simulink subsystem "Day2_Scenario_1"  (R2024a)
settings: Solver=VariableStepAuto  StartTime=0.0  StopTime=10.0  RelTol=1e-3
libraries: CarMaker4SL x2
settings Model: Creator=junhyung.cha  LastModifiedBy=User

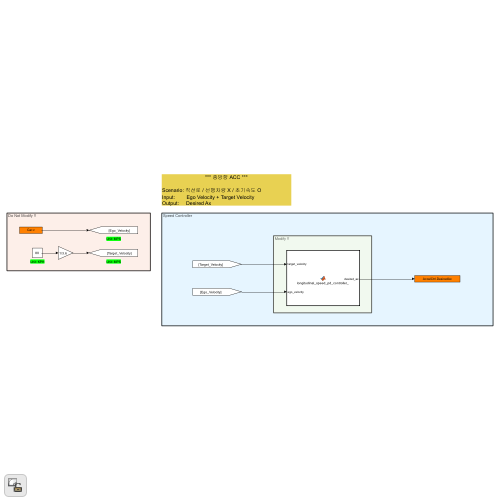
[thumbnail: Simulink's stored preview of the top-level diagram]
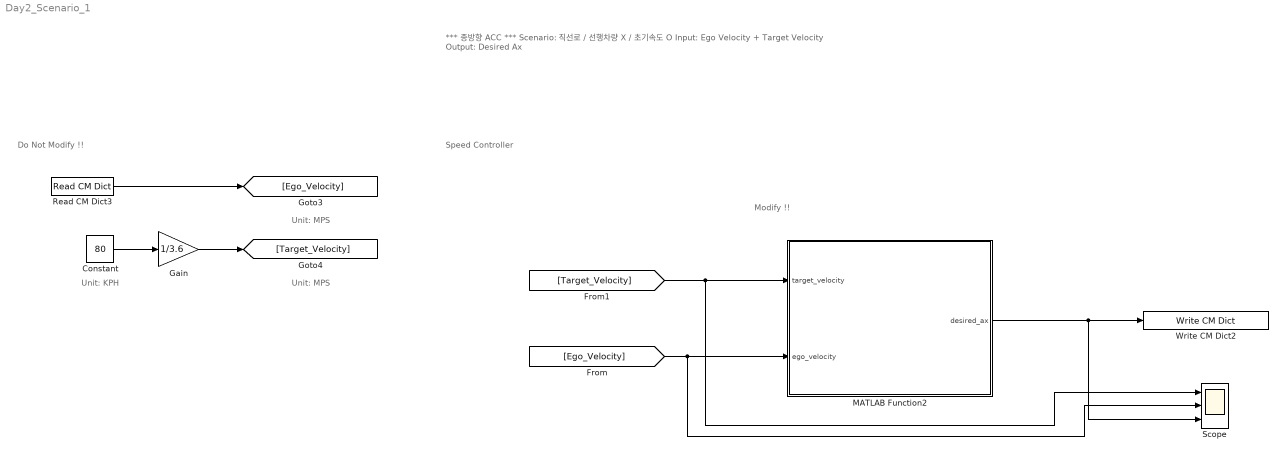
== system Day2_Scenario_1 ==
  note: Unit: KPH
  note: *** 종방향 ACC ***
      |
      | Scenario: 직선로 / 선행차량 X / 초기속도 O
      | Input: Ego Velocity + Target Velocity
      | Output: Desired Ax
  note: Do Not Modify !!
  note: Modify !!
  note: Speed Controller
  note: Unit: MPS
  note: Unit: MPS
  Constant : Constant  Value=80
  Gain : Gain  Gain=1/3.6
  MATLAB Function2 : MATLAB Function  TreatAsAtomicUnit=on
  Read CM Dict3 : CarMaker4SL/Read CM Dict  xname=Car.v  xsync=off  xstime=Inherited
  Scope : Scope  NumInputPorts=3
  Write CM Dict2 : CarMaker4SL/Write CM Dict  xname=AccelCtrl.DesiredAx  xsync=off
  wires:
  MATLAB Function2/1(desired_ax) -> Write CM Dict2/1, Scope/3
  [Target_Velocity] -> MATLAB Function2/1(target_velocity), Scope/1
  Constant/1 -> Gain/1
  [Ego_Velocity] -> MATLAB Function2/2(ego_velocity), Scope/2
  Read CM Dict3/1 -> [Ego_Velocity]
  Gain/1 -> [Target_Velocity]

== matlab function Day2_Scenario_1/MATLAB Function2 ==
  settings: updateMethod=DISCRETE  sampleTime=0.05
  data: target_velocity input; desired_ax output; ego_velocity input
function desired_ax = longitudinal_speed_pd_controller_(target_velocity, ego_velocity)
    desired_ax = 0;

    % longitudinal_speed_pd_controller_  PD speed controller for ACC
%   Inputs:
%     target_velocity - 목표 속도 [m/s]
%     ego_velocity    - 현재 자차 속도 [m/s]
%   Output:
%     desired_ax      - 원하는 종방향 가속도 [m/s^2]

  %#codegen
  persistent Kp Kd dt prev_error
  if isempty(Kp)
    % — PD 게인 설정 (필요에 따라 조정하세요) —
    Kp = 1.4;    % 비례 이득
    Kd = 0.001;    % 미분 이득
    % — 제어 업데이트 주기 (Simulink 샘플타임과 동일하게) —
    dt = 0.1;    % [s]
    % — previous error 초기화 —
    prev_error = target_velocity - ego_velocity;
  end

  % 1) 속도 오차
  error = target_velocity - ego_velocity;
  % 2) 오차 변화율 (미분항)
  derivative = (error - prev_error) / dt;
  % 3) PD 제어 법칙
  desired_ax = Kp * error + Kd * derivative;
  % 4) 이전 오차 갱신
  prev_error = error;
end
